simulink model "untitled"  (R2024b)
settings: Solver=FixedStepAuto  StartTime=0.0  StopTime=inf  FixedStep=0.001  RelTol=1e-3  EnableMultiTasking=on
libraries: simulink x2, stm32f4xxblockslib x1
settings Model: STM32="{\"AnalogInput\":{\"ID\":\"untitled:1\"}}"  PacingRate=0.110000  Creator=User  LastModifiedBy=User
settings OptimizationCC: EnhancedBackFolding=on  PassReuseOutputArgsAs=Individual arguments  ZeroExternalMemoryAtStartup=off  ZeroInternalMemoryAtStartup=off  MaxStackSize=512  OptimizeBlockOrder=speed  DifferentSizesBufferReuse=on  OptimizationCustomize=off  EfficientTunableParamExpr=on
settings DebuggingCC: ParameterTunabilityLossMsg=error
settings HardwareCC: ProdBitPerPointer=32  ProdBitPerSizeT=32  ProdBitPerPtrDiffT=32  ProdLargestAtomicInteger=Long  ProdLargestAtomicFloat=Double  ProdWordSize=32  ProdLongLongMode=on  ProdHWDeviceType=ARM Compatible->ARM Cortex-M
settings SFSimCC: MATLABDynamicMemAlloc=off  SimHardwareAcceleration=off
settings RTWCC: Description=Embedded Coder  SystemTargetFile=ert.tlc  HardwareBoard=STM32G4xx Based  TemplateMakefile=ert_default_tmf  Toolchain=GNU Tools for ARM Embedded Processors
settings CodeAppCC: ForceParamTrailComments=on  IgnoreCustomStorageClasses=off  OperatorAnnotations=on  SimulinkDataObjDesc=on  SFDataObjDesc=on  InsertBlockDesc=on
settings ERTTargetCC: TargetLangStandard=C99 (ISO)  CodeReplacementLibrary=ARM Cortex-M  ExtModeTransport=3  ExtModeStaticAlloc=on  ExtModeStaticAllocSize=2048  ExtModeMexFile=ext_xcp  ExtModeIntrfLevel=Level2 - Open  InlinedParameterPlacement=Hierarchical  DynamicArrayContainerType=coder::array

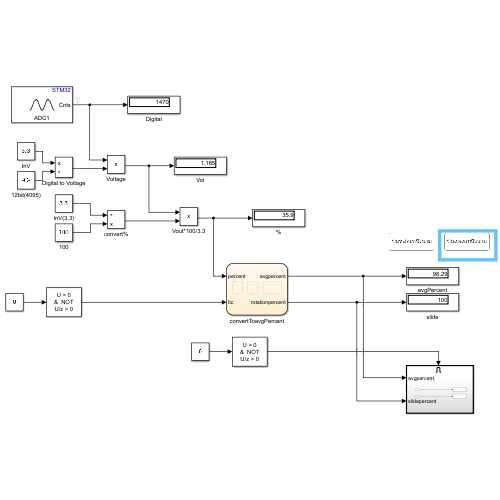
[thumbnail: Simulink's stored preview of the top-level diagram]
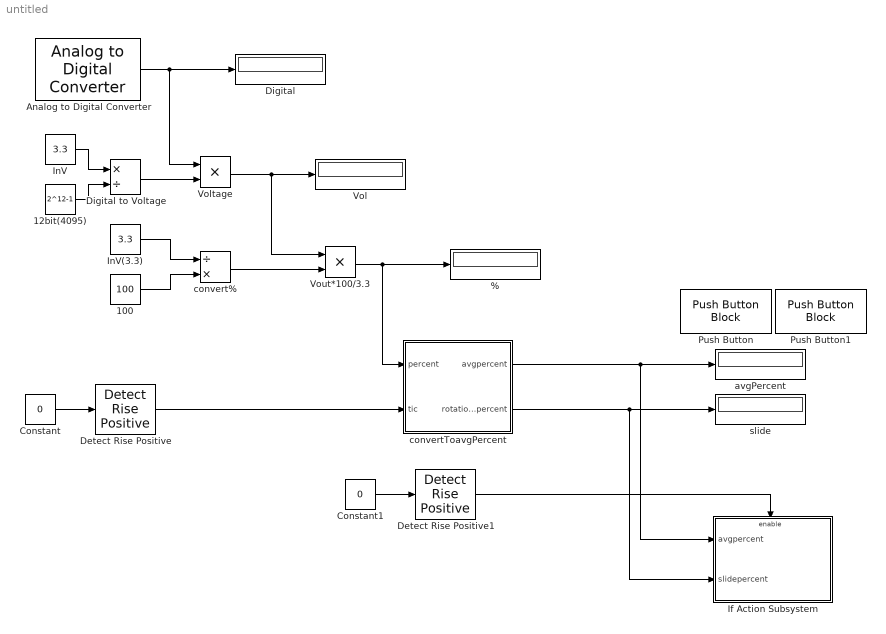
== system untitled ==
  % : Display
  100 : Constant  Value=100
  12bit(4095) : Constant  Value=2^12-1
  Analog to Digital Converter : stm32f4xxblockslib/Analog to Digital Converter  ADCModule=ADC1  ConversionGroup=Regular  TriggerMode=Trigger and read  NumberOfConversions=1  EnableBufferConv=off  BufferLength=1  OutputStatus=off  SampleTime=-1  EnableSimPort=off  hoistedMaskSrc=ECSoC/ECSimCodegen/Analog to Digital Converter
  Constant : Constant  Value=0
  Constant1 : Constant  Value=0
  Detect Rise Positive : simulink/Logic and Bit Operations/Detect Rise Positive  vinit=0  OutDataTypeStr=boolean
  Detect Rise Positive1 : simulink/Logic and Bit Operations/Detect Rise Positive  vinit=0  OutDataTypeStr=boolean
  Digital : Display
  Digital to Voltage : Product  Inputs=*/
  If Action Subsystem : Subsystem  TreatAsAtomicUnit=on
  InV : Constant  Value=3.3
  InV(3.3) : Constant  Value=3.3
  Push Button : PushButtonBlock  ButtonText=ปุ่มหล่อเท่นิรนาม  OffValue=0.000000
  Push Button1 : PushButtonBlock  ButtonText=ปุ่มสุดสวยนิรนาม  OffValue=0.000000
  Vol : Display
  Voltage : Product
  Vout*100/3.3 : Product
  avgPercent : Display
  convert% : Product  Inputs=/*
  convertToavgPercent : Stateflow chart  TreatAsAtomicUnit=on
  slide : Display
  wires:
  Analog to Digital Converter/1 -> Voltage/1, Digital/1
  Constant/1 -> Detect Rise Positive/1
  InV/1 -> Digital to Voltage/1
  12bit(4095)/1 -> Digital to Voltage/2
  Digital to Voltage/1 -> Voltage/2
  Voltage/1 -> Vout*100/3.3/1, Vol/1
  InV(3.3)/1 -> convert%/1
  100/1 -> convert%/2
  convert%/1 -> Vout*100/3.3/2
  Vout*100/3.3/1 -> convertToavgPercent/1(percent), %/1
  Detect Rise Positive/1 -> convertToavgPercent/2(tic)
  Constant1/1 -> Detect Rise Positive1/1
  convertToavgPercent/2(rotationpercent) -> If Action Subsystem/2(slidepercent), slide/1
  convertToavgPercent/1(avgpercent) -> If Action Subsystem/1(avgpercent), avgPercent/1
  Detect Rise Positive1/1 -> If Action Subsystem/Enable

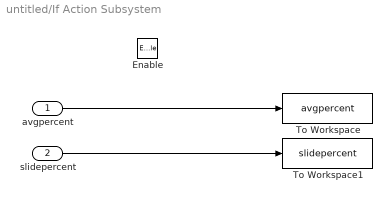
== system untitled/If Action Subsystem ==
  avgpercent : Inport
  slidepercent : Inport  Port=2
  Enable : EnablePort
  To Workspace : ToWorkspace  VariableName=avgpercent  SampleTime=-1
  To Workspace1 : ToWorkspace  VariableName=slidepercent  SampleTime=-1
  wires:
  avgpercent/1 -> To Workspace/1
  slidepercent/1 -> To Workspace1/1

== stateflow chart untitled/convertToavgPercent ==
  state start
    entry:
    contain = 0;
    counting = 1000;
    time = 0;
    rotationpercent = -10;
  state reset
    entry:
    contain = 0;
    counting = 1000;
    time = 0;
  state get1000value
    during:
    time = time+0.001;
    contain = contain+percent;
    exit:
    avgpercent = contain/counting;
    rotationpercent = rotationpercent + 10;
  (default) -> start
  start -> reset
  reset -> get1000value : [tic == 1]
  get1000value -> reset : [time >= 1]
  data: percent input; tic input; avgpercent output; time local; contain local; counting local; rotationpercent output
